simulink model "simulink_discrete_2_R2021a"  (R2023b)
settings: Solver=ode23  StartTime=0.0  StopTime=0.7  FixedStep=T1  MaxStep=1E-5  RelTol=1e-3  EnableMultiTasking=on
undefined symbols (not defined in the file): Ts
libraries: cstblocks x10
settings Model: Creator=Koldo  LastModifiedBy=chris
settings SolverCC: ShapePreserveControl=EnableAll  ZeroCrossAlgorithm=Adaptive  AlgebraicLoopSolver=TrustRegion  PositivePriorityOrder=on  AutoInsertRateTranBlk=on  InsertRTBMode=Never (minimum delay)
settings DataIOCC: LimitDataPoints=on  SaveFormat=Array  SignalLoggingSaveFormat=ModelDataLogs  ReturnWorkspaceOutputs=off
settings OptimizationCC: ExpressionDepthLimit=2147483647  LifeSpan=inf
settings DebuggingCC: UnderspecifiedInitializationDetection=Classic  MergeDetectMultiDrivingBlocksExec=none  IgnoredZcDiagnostic=none  SolverPrmCheckMsg=warning  FcnCallInpInsideContextMsg=warning  UnconnectedInputMsg=warning  UnconnectedOutputMsg=warning  UnconnectedLineMsg=warning  StateNameClashWarn=warning  SFUnexpectedBacktrackingDiag=warning  SFNoUnconditionalDefaultTransitionDiag=warning  SFExecutionAtInitializationDiag=none  ArithmeticOperatorsInVariantConditions=warning
settings HardwareCC: ProdBitPerPointer=32  ProdBitPerSizeT=32  ProdBitPerPtrDiffT=32  ProdLargestAtomicFloat=None  ProdIntDivRoundTo=Undefined  ProdEndianess=Unspecified  ProdWordSize=32  ProdHWDeviceType=32-bit Generic
settings ModelReferenceCC: EnableRefExpFcnMdlSchedulingChecks=on  PropagateSignalLabelsOutOfModel=off
settings SFSimCC: SimUseLocalCustomCode=off  CustomCodeUndefinedFunction=UseInterfaceOnly
settings RTWCC: RTWUseLocalCustomCode=off  DLArmComputeVersion=19.05
settings CodeAppCC: StateflowObjectComments=on
settings GRTTargetCC: TargetLangStandard=C89/C90 (ANSI)  CombineOutputUpdateFcns=off  GRTInterface=on
settings ConfigComp: CovMetricSettings=dw  CovSaveCumulativeToWorkspaceVar=on  CovSaveSingleToWorkspaceVar=on  CovExternalEMLEnable=off

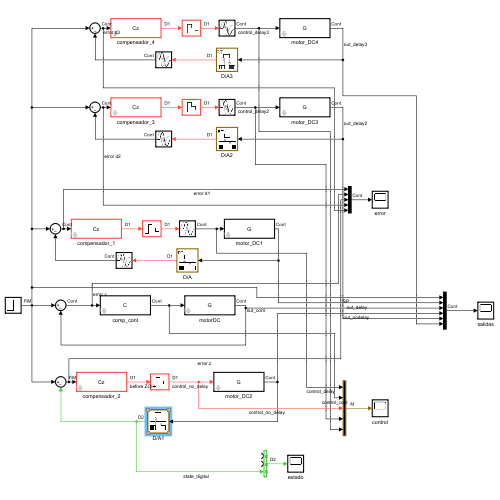
[thumbnail: Simulink's stored preview of the top-level diagram]
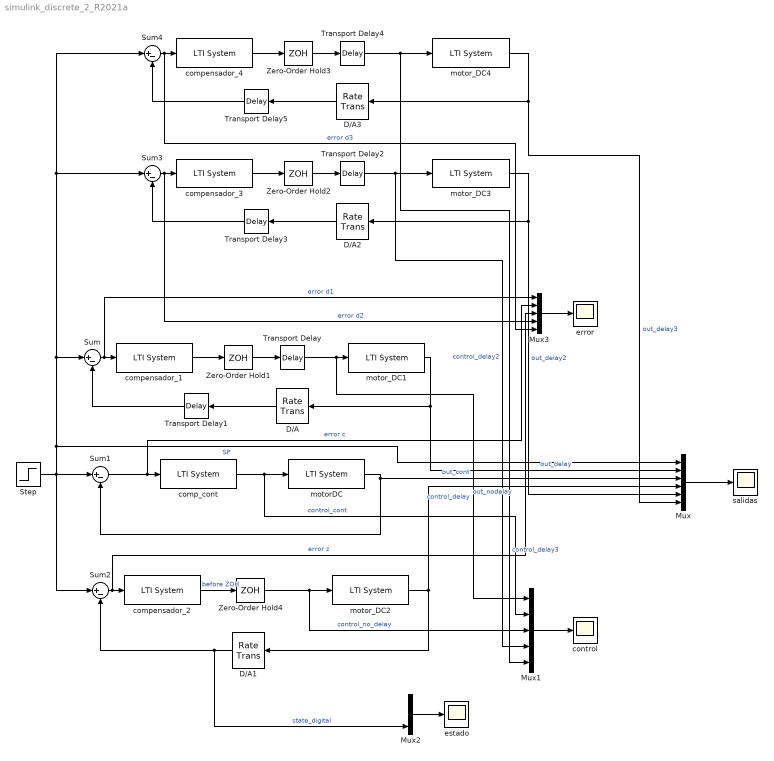
== system simulink_discrete_2_R2021a ==
  D/A : RateTransition  Priority=0  Integrity=off  Deterministic=off  OutPortSampleTime=Ts
  D/A1 : RateTransition  OutPortSampleTime=0.01
  D/A2 : RateTransition  Priority=0  Integrity=off  Deterministic=off  OutPortSampleTime=Ts
  D/A3 : RateTransition  Priority=0  Integrity=off  Deterministic=off  OutPortSampleTime=Ts
  Mux : Mux  Inputs=6
  Mux1 : Mux  Inputs=5
  Mux2 : Mux  Inputs=3
      settings: DisplayOption=signals
  Mux3 : Mux  Inputs=5
  Step : Step  Time=0.1  After=pi/2  SampleTime=0
  Sum{,1..4} (5 alike) : Sum  Inputs=|+-
  Transport Delay : TransportDelay  DelayTime=0.1*Ts
  Transport Delay1 : TransportDelay  DelayTime=0.1*Ts
  Transport Delay2 : TransportDelay  DelayTime=0.5*Ts
  Transport Delay3 : TransportDelay  DelayTime=0.5*Ts
  Transport Delay4 : TransportDelay  DelayTime=1.5*Ts
  Transport Delay5 : TransportDelay  DelayTime=1.5*Ts
  Zero-Order Hold{1..4} (4 alike) : ZeroOrderHold  SampleTime=Ts
  comp_cont : cstblocks/LTI System  sys=C  IC=[]  PadeOrder=0
  compensador_{1..4} (4 alike) : cstblocks/LTI System  Priority=1  sys=Cz  IC=[]  PadeOrder=0
  control : Scope
  error : Scope
  estado : Scope
  motorDC : cstblocks/LTI System  sys=G  IC=[]  PadeOrder=0
  motor_DC{1..4} (4 alike) : cstblocks/LTI System  sys=G  IC=[]  PadeOrder=0
  salidas : Scope
  wires:
  Sum/1 -> Mux3/1, compensador_1/1  "error d1"
  compensador_1/1 -> Zero-Order Hold1/1
  Sum1/1 -> Mux3/2, comp_cont/1  "error c"
  motorDC/1 -> Sum1/2, Mux/3  "out_cont"
  comp_cont/1 -> motorDC/1, Mux1/2  "control_cont"
  Mux/1 -> salidas/1
  Step/1 -> Sum4/1, Sum3/1, Sum/1, Mux/1, Sum1/1, Sum2/1  "SP"
  Sum2/1 -> Mux3/3, compensador_2/1  "error z"
  Zero-Order Hold4/1 -> motor_DC2/1, Mux1/3  "control_no_delay"
  Mux1/1 -> control/1
  motor_DC1/1 -> D/A/1, Mux/2  "out_delay"
  compensador_2/1 -> Zero-Order Hold4/1  "before ZOH"
  Zero-Order Hold1/1 -> Transport Delay/1
  Transport Delay/1 -> motor_DC1/1, Mux1/1  "control_delay"
  Transport Delay1/1 -> Sum/2
  D/A/1 -> Transport Delay1/1
  motor_DC2/1 -> D/A1/1, Mux/4  "out_nodelay"
  Mux2/1 -> estado/1
  D/A1/1 -> Sum2/2, Mux2/3  "state_digital"
  Mux3/1 -> error/1
  Zero-Order Hold2/1 -> Transport Delay2/1
  motor_DC3/1 -> Mux/5, D/A2/1  "out_delay2"
  Transport Delay3/1 -> Sum3/2
  Transport Delay2/1 -> Mux1/4, motor_DC3/1  "control_delay2"
  compensador_3/1 -> Zero-Order Hold2/1
  Sum3/1 -> Mux3/4, compensador_3/1  "error d2"
  D/A2/1 -> Transport Delay3/1
  Transport Delay5/1 -> Sum4/2
  D/A3/1 -> Transport Delay5/1
  compensador_4/1 -> Zero-Order Hold3/1
  Transport Delay4/1 -> Mux1/5, motor_DC4/1  "control_delay3"
  Zero-Order Hold3/1 -> Transport Delay4/1
  Sum4/1 -> Mux3/5, compensador_4/1  "error d3"
  motor_DC4/1 -> Mux/6, D/A3/1  "out_delay3"
